simulink library "Methanol_Synthasis"  (R2023a)
settings: Solver=VariableStepAuto  StartTime=0.0  StopTime=10.0  RelTol=1e-3
settings Model: Creator=mekala.suresh  LastModifiedBy=andres.lucht
settings OptimizationCC: ReuseModelBlockBuffer=off

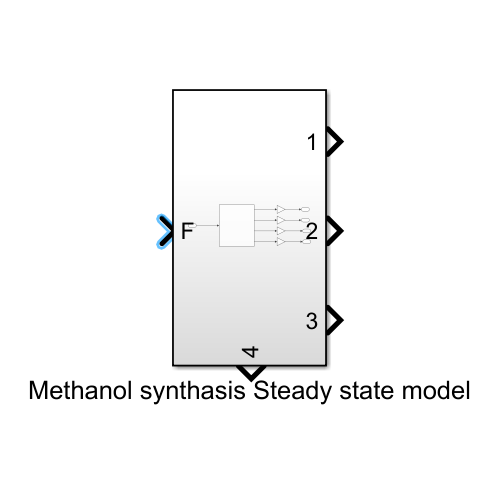
[thumbnail: Simulink's stored preview of the top-level diagram]
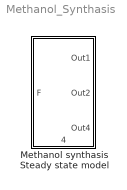
== system Methanol_Synthasis ==
  Methanol synthasis Steady state model : Subsystem
      settings: PortSchema="{\"entries\":[{\"content\":{\"sides\":[{\"content\":{\"connectorIds\":[\"In1\"]},\"type\":\"ConnectorPlacement.EquallySpacedRectSide\",\"uuid\":\"9165e5ac-d4f0-4995-b309-c48bdcb74d3d\"},{\"content\":{\"connectorIds\":[\"Out1\",\"Out2\",\"Out3\"],\"side\":\"RIGHT\"},\"type\":\"ConnectorPlacement.EquallySpacedRectSide\",\"uuid\":\"5a0de348-0c76-459c-b60c-1ab4fc3ad594\"},{\"content\":{\"connectorIds\":[],\"side\":\"TOP\"},\"type\":\"ConnectorPlacement.EquallySpacedRectSide\",\"uuid\":\"71084b33-66f2-4ada-9c37-aaca34906471\"},{\"content\":{\"connectorIds\":[\"Out4\"],\"side\":\"BOTTOM\"},\"type\":\"ConnectorPlacement.EquallySpacedRectSide\",\"uuid\":\"357b4987-b5bb-450e-8f17-0d415a5fb536\"}]},\"type\":\"ConnectorPlacement.EquallySpacedConnector\",\"uuid\":\"cf3a3340-22fe-4062-a4a2-417676329b31\"}],\"packageUris\":[\"http://schema.mathworks.com/mf0/Connector/R2020b\"],\"version\":\"1.0\"}"

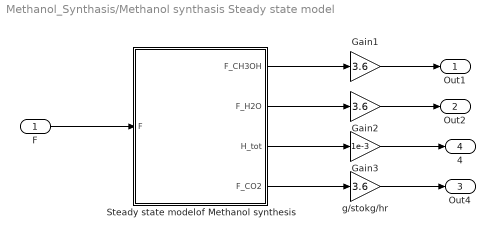
== system Methanol_Synthasis/Methanol synthasis Steady state model ==
  F : Inport
  Gain1 : Gain  Gain=3.6
  Gain2 : Gain  Gain=3.6
  Gain3 : Gain  Gain=1e-3
  Steady state modelof Methanol synthesis : MATLAB Function  TreatAsAtomicUnit=on
  g/stokg/hr : Gain  Gain=3.6
  Out1 : Outport
  Out2 : Outport  Port=2
  Out4 : Outport  Port=3
  4 : Outport  Port=4
  wires:
  Steady state modelof Methanol synthesis/1(F_CH3OH) -> Gain1/1
  Gain1/1 -> Out1/1
  Steady state modelof Methanol synthesis/3(H_tot) -> Gain3/1
  F/1 -> Steady state modelof Methanol synthesis/1(F)
  Steady state modelof Methanol synthesis/2(F_H2O) -> Gain2/1
  Gain2/1 -> Out2/1
  Gain3/1 -> 4/1
  Steady state modelof Methanol synthesis/4(F_CO2) -> g/stokg/hr/1
  g/stokg/hr/1 -> Out4/1

== matlab function Methanol_Synthasis/Methanol synthasis Steady state model/Steady state modelof Methanol synthesis ==
  data: F input; F_CH3OH output; F_H2O output; H_tot output; F_CO2 output
% Copyright 2023 DECHEMA e.V., Theodor-Heuss-Allee 25, 60486 Frankfurt, Germany (https://dechema.de)
    % Contact: Andres Lucht Uribe
    % Developer: Suresh Mekala
    % Project H2Mare: https://www.wasserstoff-leitprojekte.de/projects/h2mare

function [F_CH3OH,F_H2O,H_tot,F_CO2] = fcn(F)
% CO2 + 3H2 ⇋ CH3OH + H2O   _____1
% CO + 2H2 ⇋ CH3OH          _____2
% CO + H2O ⇋ CO2 + H2       _____3



%Reactents   %Products
    % H2         CH3OH
    % CO2        H2O 
% Reactor dimentions
D = 0.5;
L = 1.5;
V = (pi/4)*D^2*L;

% Tubular reactor volume must be specified
% Mass of the catalyst in kg
m_cat = 100 ; 
% Initial conditions
T = 250 + 273;                                                  %K % Operating temererature are between 210-250°C as specified in the litarature
P = 50 ;                                                        %bar
R = 8.31 ;                                                      %j/mol K
% molar fractions
xCO = 0.15;xH2O = 0;xCH3OH = 0;xH2=0.7;xCO2 = 0.15; xInert = 0;
% number of moles in the volume

n = (P*V)/(R*T);
C_COin = (n*xCO)/V; 
C_H2in = (n*xH2)/V;
C_CO2in = (n*xCO2)/V;
C_H2Oin = (n*xH2O)/V;
C_CH3OHin = (n*xCH3OH)/V;

% partial pressures
p_CO=P*xCO;
p_CO2=P*xCO2;
p_H2O=P*xH2O;
p_H2=P*xH2;
p_CH3OH=P*xCH3OH;

% reaction rate constants
%p = A*exp(B/RT);
k1 = 0.4999*exp(17197/(R*T));
k2 = 6.62e-11*exp(124119/(R*T));
K_WH = 3453.38;
K_H2 = 1.07*exp(36696/(R*T));
K_H2O = 1.22e10*exp(-94765/(R*T));
K1_eq = 2.391e-13 * exp(98388/(R*T));
K3_eq = 2.554e-11 * exp(58705/(R*T));


N1 = k1*p_CO2*(1-((p_CH3OH*p_H2O)/(K1_eq*p_CO2*p_H2^3)));
D1 = (1+(K_WH*p_H2O/p_H2)+sqrt(K_H2*p_H2)+(K_H2O*p_H2O))^3;

r_CH3OH = N1/D1;

N2 = k2*p_CO2*(1-(K3_eq*((p_H2O*p_CO)/(p_CO2*p_H2))));
D2 = 1 + ((K_WH*p_H2O)/p_H2)+sqrt(K_H2*p_H2)+(K_H2O*p_H2O);

r_RWGS = N2/D2;
R1 = 0;
R2 = r_CH3OH*m_cat;
R3= r_RWGS * m_cat;

% Outlet Concentrations

C_CO = C_COin-((R1+R3)*(V/F));
C_H2 = C_H2in+(((2*R1)+(3*R2)-R3)*(V/F));
C_CO2 = C_CO2in + ((R2-R3)*(V/F));
C_H2O = C_H2Oin - ((-R2+R3)*(V/F));
C_CH3OH = C_CH3OHin-((-R1-R3)*(V/F));

% Outlet flow rates
F_CO = C_CO*F;
F_H2 = C_H2*F;
F_CO2 = C_CO2*F;
F_H2O = C_H2O*F;
F_CH3OH = C_CH3OH*F;
%Heat Generated computation 

% Define the temperature-dependent enthalpies of reaction (kJ/mol)
deltaH1 =(-49.4 + 0.252*T);                                 % CO2 + 3H2 ⇋ CH3OH + H2O
deltaH2 =(-90.6 + 0.187*T);                                 % CO + 2H2 ⇋ CH3OH
deltaH3 =(41.0 - 0.055*T);                                  % CO + H2O ⇋ CO2 + H2  while the reaction enthalpiy here it is considered is for H2

nu1 = 1; % CO2 + 3H2 ⇋ CH3OH + H2O
nu2 = 1; % CO + 2H2 ⇋ CH3OH
nu3 = -1; % CO + H2O ⇋ CO2 + H2

Q1 = nu1 * deltaH1 * F_CH3OH;
Q2 = nu2 * deltaH2 * F_CH3OH;
Q3 = nu3 * deltaH3 * F_H2;
H_tot = Q1 + Q2 + Q3;
